simulink model "sim_env_falling_leaf"  (R2023b)
settings: Solver=ode113  StartTime=0.0  StopTime=20  RelTol=1e-3
model workspace (MAT data in the model file):
  ail_0 = -0.0765
settings Model: Creator=ac140857  LastModifiedBy=fabioschneider

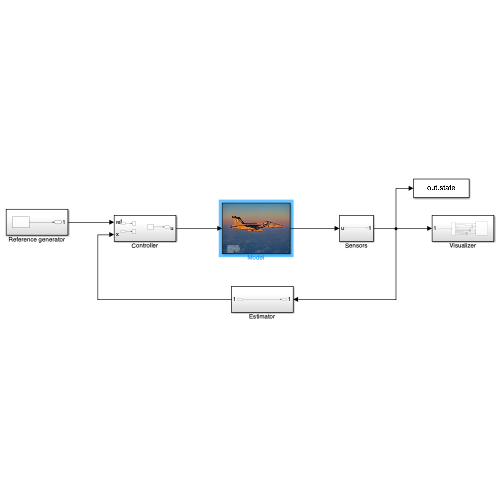
[thumbnail: Simulink's stored preview of the top-level diagram]
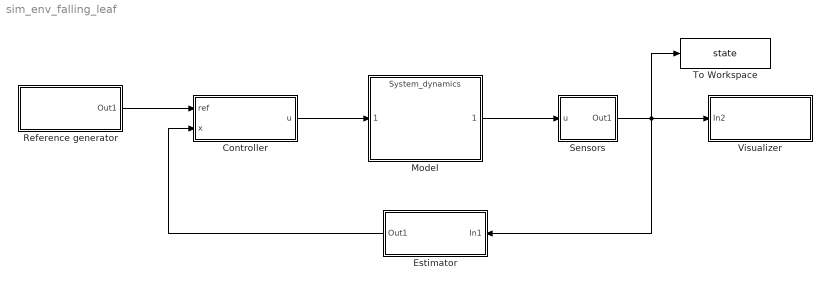
== system sim_env_falling_leaf ==
  Controller : Subsystem
  Estimator : Subsystem
  Model : ModelReference  ModelNameDialog=System_dynamics.slx  SimulationMode=Normal  ModelReferenceVersion=4.84
      mask Display: image('F-18_image Small.jpeg');
  Reference generator : Subsystem
  Sensors : Subsystem
  To Workspace : ToWorkspace  VariableName=state  SaveFormat=Timeseries  SampleTime=-1
  Visualizer : Subsystem
  wires:
  Reference generator/1(Out1) -> Controller/1(ref)
  Estimator/1(Out1) -> Controller/2(x)
  Sensors/1(Out1) -> To Workspace/1, Visualizer/1(In2), Estimator/1(In1)
  Controller/1(u) -> Model/1
  Model/1 -> Sensors/1(u)

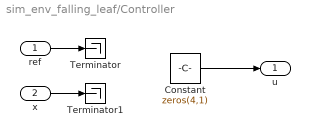
== system sim_env_falling_leaf/Controller ==
  ref : Inport
  x : Inport  Port=2
  Constant : Constant  Value=zeros(4,1)
  Terminator : Terminator
  Terminator1 : Terminator
  u : Outport
  wires:
  ref/1 -> Terminator/1
  x/1 -> Terminator1/1
  Constant/1 -> u/1

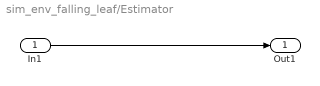
== system sim_env_falling_leaf/Estimator ==
  In1 : Inport
  Out1 : Outport
  wires:
  In1/1 -> Out1/1

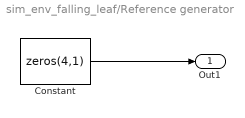
== system sim_env_falling_leaf/Reference generator ==
  Constant : Constant  Value=zeros(4,1)
  Out1 : Outport
  wires:
  Constant/1 -> Out1/1

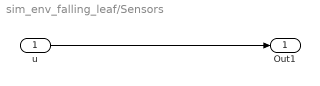
== system sim_env_falling_leaf/Sensors ==
  u : Inport
  Out1 : Outport
  wires:
  u/1 -> Out1/1

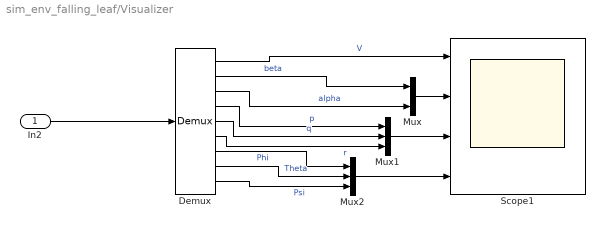
== system sim_env_falling_leaf/Visualizer ==
  In2 : Inport
  Demux : Demux  Outputs=9
  Mux : Mux  Inputs=2
  Mux1 : Mux  Inputs=3
  Mux2 : Mux  Inputs=3
  Scope1 : Scope  NumInputPorts=4
  wires:
  In2/1 -> Demux/1
  Demux/6 -> Mux1/3  "r"
  Demux/5 -> Mux1/2  "q"
  Demux/4 -> Mux1/1  "p"
  Demux/8 -> Mux2/2  "Theta"
  Demux/7 -> Mux2/1  "Phi"
  Demux/2 -> Mux/1  "beta"
  Demux/1 -> Scope1/1  "V"
  Mux/1 -> Scope1/2
  Demux/3 -> Mux/2  "alpha"
  Mux2/1 -> Scope1/4
  Demux/9 -> Mux2/3  "Psi"
  Mux1/1 -> Scope1/3
